simulink model "Day2_1_filter_design"  (R2022b)
settings: Solver=FixedStepAuto  StartTime=0.0  StopTime=10  FixedStep=0.001  RelTol=1e-3
InitFcn:
  | cutoff_freq = 10;
  | Ts = 0.001;
  | LPF1 = tf([cutoff_freq], [1 cutoff_freq]);
  | LPF1d = c2d(LPF1, Ts);
  | b = LPF1d.Numerator{1};
  | a = LPF1d.Denominator{1};
settings Model: Creator=user  LastModifiedBy=user

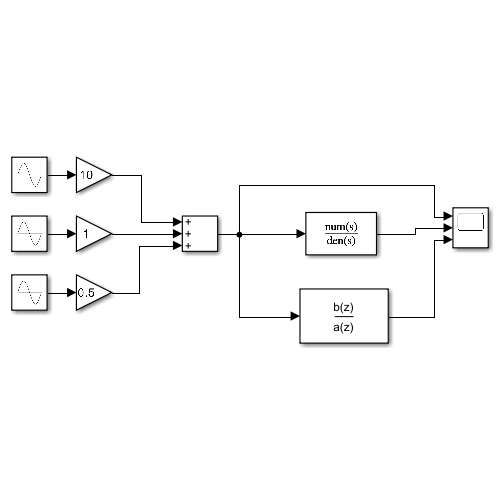
[thumbnail: Simulink's stored preview of the top-level diagram]
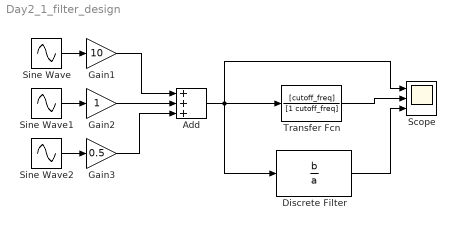
== system Day2_1_filter_design ==
  Add : Sum  Inputs=+++
  Discrete Filter : DiscreteFilter  Numerator=b  Denominator=a
  Gain1 : Gain  Gain=10
  Gain2 : Gain
  Gain3 : Gain  Gain=0.5
  Scope : Scope  NumInputPorts=3
  Sine Wave : Sin  Frequency=0.25*2*pi  SampleTime=0
  Sine Wave1 : Sin  Frequency=10*2*pi  SampleTime=0
  Sine Wave2 : Sin  Frequency=200*2*pi  SampleTime=0
  Transfer Fcn : TransferFcn  Numerator=[cutoff_freq]  Denominator=[1 cutoff_freq]
  wires:
  Sine Wave/1 -> Gain1/1
  Sine Wave1/1 -> Gain2/1
  Add/1 -> Transfer Fcn/1, Discrete Filter/1, Scope/1
  Transfer Fcn/1 -> Scope/2
  Sine Wave2/1 -> Gain3/1
  Discrete Filter/1 -> Scope/3
  Gain1/1 -> Add/1
  Gain2/1 -> Add/2
  Gain3/1 -> Add/3
